simulink model "Simulink"  (R2020b)
settings: Solver=ode45  StartTime=0.0  StopTime=1  MaxStep=0.0001  RelTol=1e-9  AbsTol=1e-9
values from neighbouring files (symbols this model uses):
  B = 0    [Main.m]
  iab_0 = [ia_0;ib_0]    [Main.m]
  Jm = 0.00027    [Main.m]
  Kii = Kpi*R/L    (= 6250)    [Main.m]
  Kiw = Jm*wn^2    [Main.m]
  Kpi = 3*L/Tsi    (= 30)    [Main.m]
  Kpw = 2*xi*Jm*wn-B    [Main.m]
  L = 0.03    [Main.m]
  lamda_m = 0.3200    (= 0.32)    [Main.m]
  np = 5    [Main.m]
  omega_0 = 0    [Main.m]
  R = 6.25    [Main.m]
  theta_0 = 0    [Main.m]
  TL1 = 0.151    [Main.m]
undefined symbols (not defined in the file or in its folder): sigbuilder_block
settings Model: Creator=sokra  LastModifiedBy=sokra
settings SolverCC: AutoScaleAbsTol=off

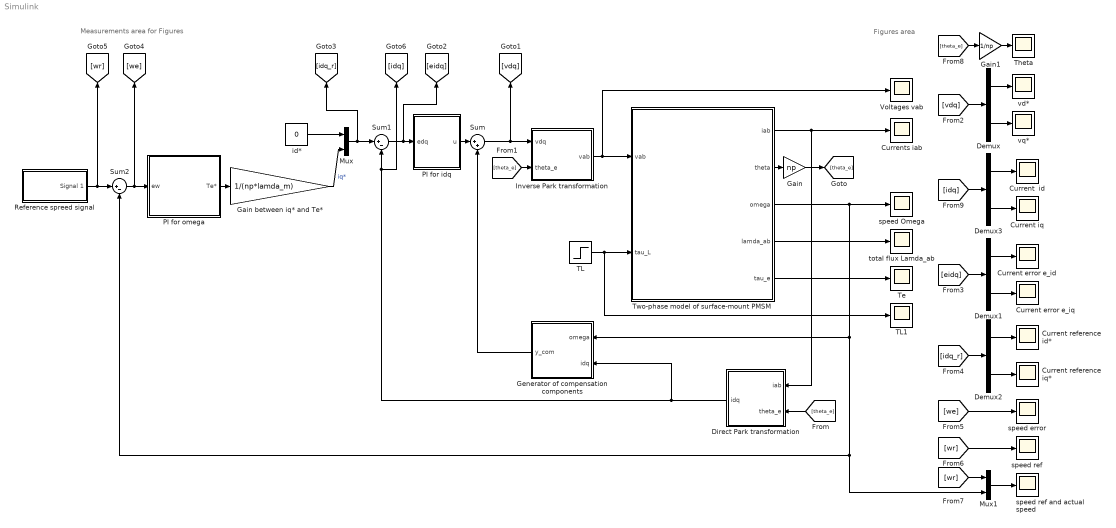
== system Simulink ==
  note: Figures area
  note: Measurements area for Figures
  Current  id : Scope
  Current error e_id : Scope
  Current error e_iq : Scope
  Current iq : Scope
  Current reference id* : Scope
  Current reference iq* : Scope
  Currents iab : Scope
  Demux{,1..3} (4 alike) : Demux  Outputs=2
  Direct Park transformation : MATLAB Function  TreatAsAtomicUnit=on
  Gain : Gain  Gain=np
  Gain between iq* and Te* : Gain  Gain=1/(np*lamda_m)
  Gain1 : Gain  Gain=1/np
  Generator of compensation components : MATLAB Function  TreatAsAtomicUnit=on
  Inverse Park transformation : MATLAB Function  TreatAsAtomicUnit=on
  Mux : Mux  Inputs=2
  Mux1 : Mux  Inputs=2
  PI for idq : Subsystem  mask{Kii_d=Kii, Kpi_d=Kpi, Kii_q=Kii, Kpi_q=Kpi}
  PI for omega : Subsystem  mask{Ki=Kiw, Kp=Kpw}
  Reference spreed signal : Subsystem  Tag=STV Subsys  LoadFcn=sigbuilder_block('load');  StartFcn=sigbuilder_block('start');  StopFcn=sigbuilder_block('stop');  ClipboardFcn=sigbuilder_block('clipboard');  mask(Sigbuilder block){tuvar=[0:10]}
      mask help: Simulink:masks:SigbuilderBlock_MD
      mask init:
      | if ~strcmp(get_param(bdroot(gcbh),'SimulationStatus'),'stopped') tuvar = sigbuilder_block('maskInit'); end
      settings: CopyFcn=sigbuilder_block('copy');  DeleteFcn=sigbuilder_block('delete');  ModelCloseFcn=sigbuilder_block('modelClose');  PreSaveFcn=sigbuilder_block('preSave');  PauseFcn=sigbuilder_block('pause');  ContinueFcn=sigbuilder_block('continue');  NameChangeFcn=sigbuilder_block('namechange');  OpenFcn=sigbuilder_block('open',[1467 209.25 550.5 359.25 ]);  CloseFcn=sigbuilder_block('close');
      mask Display: plot(0, 0, 100, 100,[2, 2, 32, 32, 2], [68, 8, 8, 68, 68],[32, 2], [38, 38], [32, 19, 2],[53, 60, 44], [32, 17, 17, 2],[16, 16, 31, 31]);txt = getActiveGroup(gcbh);text(2, 100, txt,'verticalAlignment', 'top');
  Sum : Sum  Inputs=|++
  Sum1 : Sum  Inputs=|+-
  Sum2 : Sum  Inputs=|+-
  TL : Step  Time=0.5  After=TL1  SampleTime=0
  TL1 : Scope
  Te : Scope
  Theta : Scope
  Two-phase model of surface-mount PMSM : Subsystem
  Voltages vab : Scope
  id* : Constant  Value=0
  speed Omega : Scope
  speed error : Scope
  speed ref : Scope
  speed ref and actual speed : Scope
  total flux Lamda_ab : Scope
  vd* : Scope
  vq* : Scope
  wires:
  Two-phase model of surface-mount PMSM/2(theta) -> Gain/1
  [theta_e] -> Direct Park transformation/2(theta_e)
  Direct Park transformation/1(idq) -> [idq], Sum1/2, Generator of compensation components/2(idq)
  TL/1 -> Two-phase model of surface-mount PMSM/2(tau_L), TL1/1
  Two-phase model of surface-mount PMSM/5(tau_e) -> Te/1
  Two-phase model of surface-mount PMSM/4(lamda_ab) -> total flux Lamda_ab/1
  Two-phase model of surface-mount PMSM/1(iab) -> Currents iab/1, Direct Park transformation/1(iab)
  Gain/1 -> [theta_e]
  Sum/1 -> Inverse Park transformation/1(vdq), [vdq]
  [theta_e] -> Inverse Park transformation/2(theta_e)
  Inverse Park transformation/1(vab) -> Two-phase model of surface-mount PMSM/1(vab), Voltages vab/1
  PI for idq/1(u) -> Sum/1
  Gain between iq* and Te*/1 -> Mux/2  "iq*"
  id*/1 -> Mux/1
  Generator of compensation components/1(y_com) -> Sum/2
  Sum2/1 -> PI for omega/1(ew), [we]
  Reference spreed signal/1(Signal 1) -> Sum2/1, [wr]
  Two-phase model of surface-mount PMSM/3(omega) -> Generator of compensation components/1(omega), Mux1/2, Sum2/2, speed Omega/1
  Demux/1 -> vd*/1
  Demux/2 -> vq*/1
  Sum1/1 -> PI for idq/1(edq), [eidq]
  Demux1/1 -> Current error e_id/1
  Demux1/2 -> Current error e_iq/1
  Mux/1 -> Sum1/1, [idq_r]
  Demux2/2 -> Current reference iq*/1
  Demux2/1 -> Current reference id*/1
  [idq_r] -> Demux2/1
  [vdq] -> Demux/1
  [eidq] -> Demux1/1
  [we] -> speed error/1
  [wr] -> speed ref/1
  [wr] -> Mux1/1
  Mux1/1 -> speed ref and actual speed/1
  [theta_e] -> Gain1/1
  Gain1/1 -> Theta/1
  [idq] -> Demux3/1
  Demux3/2 -> Current iq/1
  Demux3/1 -> Current  id/1
  PI for omega/1(Te*) -> Gain between iq* and Te*/1

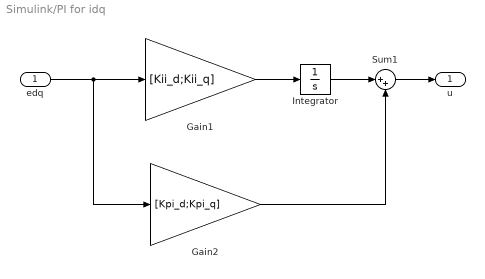
== system Simulink/PI for idq ==
  edq : Inport
  Gain1 : Gain  Gain=[Kii_d;Kii_q]
  Gain2 : Gain  Gain=[Kpi_d;Kpi_q]
  Integrator : Integrator
  Sum1 : Sum  Inputs=|++
  u : Outport
  wires:
  edq/1 -> Gain2/1, Gain1/1
  Gain1/1 -> Integrator/1
  Integrator/1 -> Sum1/1
  Gain2/1 -> Sum1/2
  Sum1/1 -> u/1

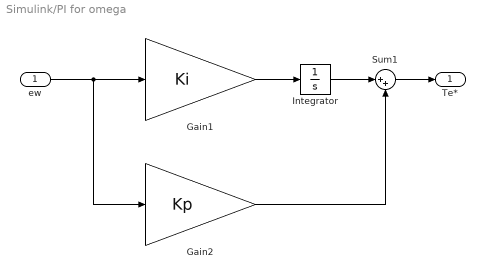
== system Simulink/PI for omega ==
  ew : Inport
  Gain1 : Gain  Gain=Ki
  Gain2 : Gain  Gain=Kp
  Integrator : Integrator
  Sum1 : Sum  Inputs=|++
  Te* : Outport
  wires:
  Sum1/1 -> Te*/1
  Gain2/1 -> Sum1/2
  Integrator/1 -> Sum1/1
  Gain1/1 -> Integrator/1
  ew/1 -> Gain1/1, Gain2/1

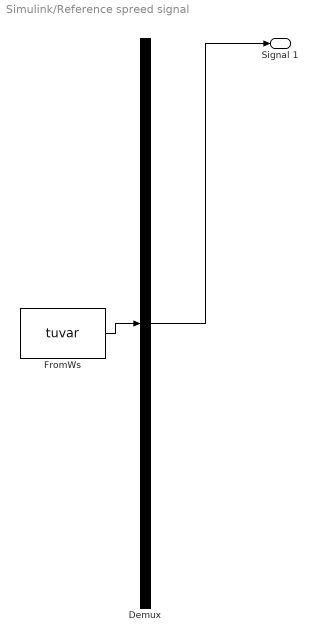
== system Simulink/Reference spreed signal ==
  Demux : Demux  Tag=STV Demux  Outputs=1
      settings: DisplayOption=none
  FromWs : FromWorkspace  Tag=STV FromWs  VariableName=tuvar
      SigBuilderData=|
      | common.afterFinalStr = 'Extrapolate'
      | common.sampleTime = 0
      | dataSet.timeRange = [0 10]
      | dataSet.name = 'Group 1'
      | sbobj.Groups.Name = 'Group 1'
      | sbobj.Groups.Signals.Name = 'Signal 1'
      | sbobj.Groups.Signals.XData = [0 0.2 6 10]
      | sbobj.Groups.Signals.YData = [0 194 194 194]
  Signal 1 : Outport  Tag=STV Outport
  wires:
  Demux/1 -> Signal 1/1
  FromWs/1 -> Demux/1

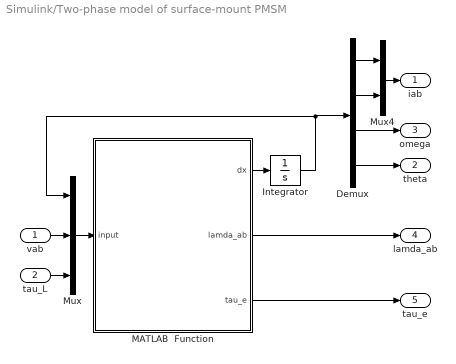
== system Simulink/Two-phase model of surface-mount PMSM ==
  vab : Inport
  tau_L : Inport  Port=2
  Demux : Demux
  Integrator : Integrator  InitialCondition=[iab_0;omega_0;theta_0]
  MATLAB  Function : MATLAB Function  TreatAsAtomicUnit=on
  Mux : Mux  Inputs=3
  Mux4 : Mux  Inputs=2
  iab : Outport
  theta : Outport  Port=2  OutDataTypeStr=double  PortDimensions=1
  omega : Outport  Port=3
  lamda_ab : Outport  Port=4
  tau_e : Outport  Port=5
  wires:
  Mux4/1 -> iab/1
  MATLAB  Function/1(dx) -> Integrator/1
  Mux/1 -> MATLAB  Function/1(input)
  Integrator/1 -> Demux/1, Mux/1
  Demux/2 -> Mux4/2
  vab/1 -> Mux/2
  MATLAB  Function/2(lamda_ab) -> lamda_ab/1
  Demux/1 -> Mux4/1
  tau_L/1 -> Mux/3
  Demux/3 -> omega/1
  Demux/4 -> theta/1
  MATLAB  Function/3(tau_e) -> tau_e/1

== matlab function Simulink/Direct Park transformation ==
  data: iab input; theta_e input; idq output
function idq = fcn(iab,theta_e)
idq = cos(theta_e+[0 -pi/2;pi/2 0])*iab;
end

== matlab function Simulink/Two-phase model of surface-mount PMSM/MATLAB  Function ==
  data: input input; dx output; lamda_ab output; R parameter; L parameter; lamda_m parameter; np parameter; Jm parameter; B parameter; tau_e output
function [dx,lamda_ab,tau_e]  = fcn(input,R, L, lamda_m, np, Jm, B)
ia=input(1);
ib=input(2);
iab=[ia;ib];
omega=input(3);
theta=input(4);
va=input(5);
vb=input(6);
vab=[va;vb];
tau_L=input(7);

%%%%%%%
C=[cos(np*theta);sin(np*theta)];
J=[0 -1;1 0];
dC=np*J*C;
%%%%%%%
dot_iab=(1/L)*(-R*iab-omega*lamda_m*dC+vab);
dot_omega=(1/Jm)*(-B*omega+lamda_m*iab'*dC-tau_L);
dot_theta=omega;
lamda_ab=L*iab+lamda_m*C;
dx = [dot_iab;dot_omega;dot_theta];
tau_e = np * iab' * J * lamda_ab;
end

== matlab function Simulink/Inverse Park transformation ==
  data: vdq input; vab output; theta_e input
function vab = fcn(vdq,theta_e)
vab = cos(theta_e+[0 pi/2;-pi/2 0])*vdq;
end

== matlab function Simulink/Generator of compensation components ==
  data: omega input; idq input; y_com output; np parameter; L parameter; lamda_m parameter
function y_com = fcn(omega,idq,np, L, lamda_m)
y_com=np*omega*[-L*idq(2);(L*idq(1)+lamda_m)];
end
